simulink model "AC_System_with_Functions"  (R2021b)
settings: Solver=ode4  StartTime=0.0  StopTime=50  FixedStep=0.05  RelTol=1e-3
values from neighbouring files (symbols this model uses):
  ActiveMode =     [AC_System_Variables.mat]
  command =     [AC_System_Variables.mat]
  Fan_Input_Modes =     [AC_System_Variables.mat]
  FanModes =     [AC_System_Variables.mat]
  RequestedMode =     [AC_System_Variables.mat]
  state =     [AC_System_Variables.mat]
undefined symbols (not defined in the file or in its folder): sigbuilder_block
settings Model: Creator=t  LastModifiedBy=t

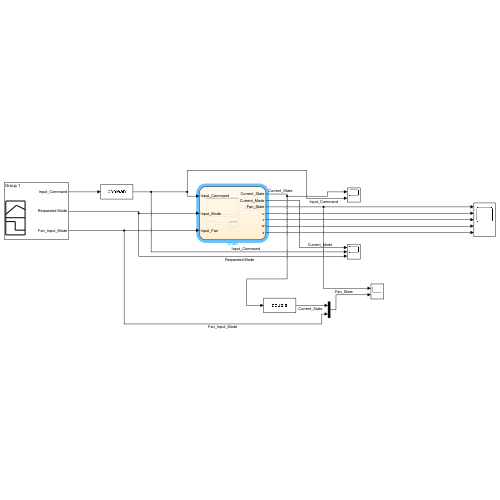
[thumbnail: Simulink's stored preview of the top-level diagram]
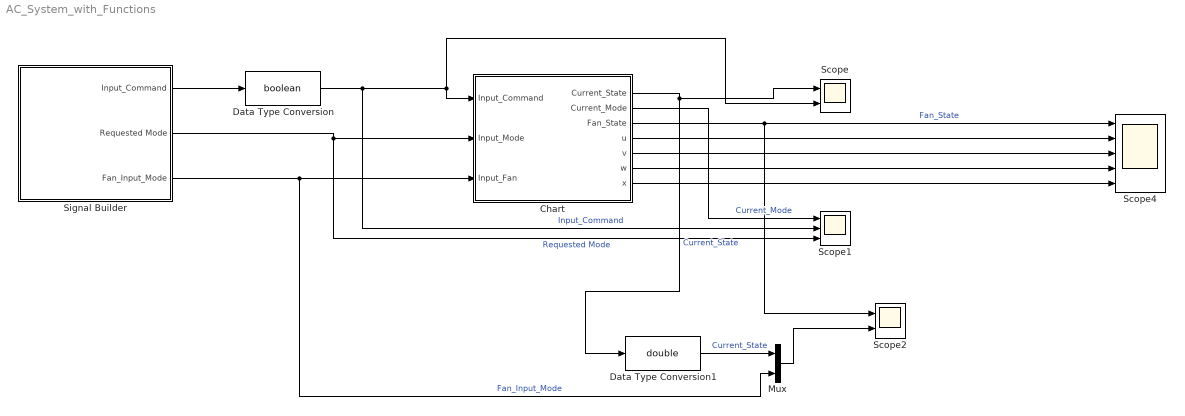
== system AC_System_with_Functions ==
  Chart : Stateflow chart  TreatAsAtomicUnit=on
  Data Type Conversion : DataTypeConversion  OutDataTypeStr=boolean
  Data Type Conversion1 : DataTypeConversion  OutDataTypeStr=double
  Mux : Mux  Inputs=2
  Scope : Scope  NumInputPorts=2
  Scope1 : Scope  NumInputPorts=3
  Scope2 : Scope  NumInputPorts=2
  Scope4 : Scope  NumInputPorts=5
  Signal Builder : Subsystem  Tag=STV Subsys  LoadFcn=sigbuilder_block('load');  StartFcn=sigbuilder_block('start');  StopFcn=sigbuilder_block('stop');  ClipboardFcn=sigbuilder_block('clipboard');  mask(Sigbuilder block){tuvar=[0:10]}
      mask help: Simulink:masks:SigbuilderBlock_MD
      mask init:
      | if ~strcmp(get_param(bdroot(gcbh),'SimulationStatus'),'stopped') tuvar = sigbuilder_block('maskInit'); end
      settings: CopyFcn=sigbuilder_block('copy');  DeleteFcn=sigbuilder_block('delete');  ModelCloseFcn=sigbuilder_block('modelClose');  PreSaveFcn=sigbuilder_block('preSave');  PauseFcn=sigbuilder_block('pause');  ContinueFcn=sigbuilder_block('continue');  NameChangeFcn=sigbuilder_block('namechange');  OpenFcn=sigbuilder_block('open',[5.4 30 1141.2 522.6 ]);  CloseFcn=sigbuilder_block('close');
      mask Display: plot(0, 0, 100, 100,[2, 2, 32, 32, 2], [68, 8, 8, 68, 68],[32, 2], [38, 38], [32, 19, 2],[53, 60, 44], [32, 17, 17, 2],[16, 16, 31, 31]);txt = getActiveGroup(gcbh);text(2, 100, txt,'verticalAlignment', 'top');
  wires:
  Signal Builder/1(Input_Command) -> Data Type Conversion/1
  Data Type Conversion/1 -> Scope1/2, Scope/2, Chart/1(Input_Command)  "Input_Command"
  Signal Builder/2(Requested Mode) -> Scope1/3, Chart/2(Input_Mode)  "Requested Mode"
  Chart/2(Current_Mode) -> Scope1/1  "Current_Mode"
  Chart/1(Current_State) -> Data Type Conversion1/1, Scope/1  "Current_State"
  Chart/3(Fan_State) -> Scope2/1, Scope4/1  "Fan_State"
  Signal Builder/3(Fan_Input_Mode) -> Mux/2, Chart/3(Input_Fan)  "Fan_Input_Mode"
  Mux/1 -> Scope2/2
  Data Type Conversion1/1 -> Mux/1  "Current_State"
  Chart/5(v) -> Scope4/3
  Chart/4(u) -> Scope4/2
  Chart/6(w) -> Scope4/4
  Chart/7(x) -> Scope4/5

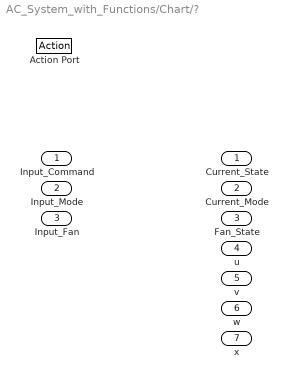
== system AC_System_with_Functions/Chart/? ==
  Input_Command : Inport
  Input_Mode : Inport  Port=2
  Input_Fan : Inport  Port=3
  Action Port : ActionPort
      settings: CopyFcn=Stateflow.SLINSF.SimulinkMan.removeBlockPreDeleteFcn  PreDeleteFcn=Stateflow.SLINSF.SimulinkMan.unsafePredeleteFcn
  Current_State : Outport
  Current_Mode : Outport  Port=2
  Fan_State : Outport  Port=3
  u : Outport  Port=4
  v : Outport  Port=5
  w : Outport  Port=6
  x : Outport  Port=7

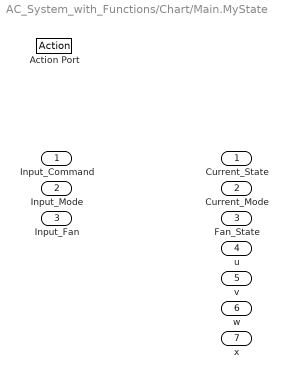
== system AC_System_with_Functions/Chart/Main.MyState ==
  Input_Command : Inport
  Input_Mode : Inport  Port=2
  Input_Fan : Inport  Port=3
  Action Port : ActionPort
      settings: CopyFcn=Stateflow.SLINSF.SimulinkMan.removeBlockPreDeleteFcn  PreDeleteFcn=Stateflow.SLINSF.SimulinkMan.unsafePredeleteFcn
  Current_State : Outport
  Current_Mode : Outport  Port=2
  Fan_State : Outport  Port=3
  u : Outport  Port=4
  v : Outport  Port=5
  w : Outport  Port=6
  x : Outport  Port=7

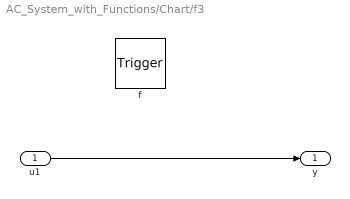
== system AC_System_with_Functions/Chart/f3 ==
  u1 : Inport  OutDataTypeStr=double  PortDimensions=1
  f : TriggerPort  TriggerType=function-call  VariantControl=(inherit)
      settings: CopyFcn=Stateflow.SLINSF.SimulinkMan.removeBlockPreDeleteFcn  PreDeleteFcn=Stateflow.SLINSF.SimulinkMan.unsafePredeleteFcn
  y : Outport
  wires:
  u1/1 -> y/1

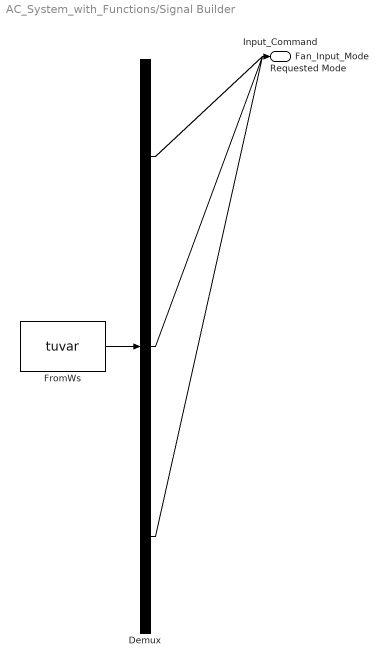
== system AC_System_with_Functions/Signal Builder ==
  Demux : Demux  Tag=STV Demux  Outputs=3
      settings: DisplayOption=none
  FromWs : FromWorkspace  Tag=STV FromWs  VariableName=tuvar
      SigBuilderData=|
      | common.afterFinalStr = 'Extrapolate'
      | common.sampleTime = 0
      | dataSet.timeRange = [0 50]
      | dataSet.name = 'Group 1'
      | sbobj.Groups.Name = 'Group 1'
      | sbobj.Groups.Signals(1).Name = 'Input_Command'
      | sbobj.Groups.Signals(1).XData = [0 1.3 1.3 33.5 33.5 36.5 36.5 38 38 40.2 40.2 47 47 50]
      | sbobj.Groups.Signals(1).YData = [0 0 1 1 0 0 1 1 0 0 1 1 0 0]
      | sbobj.Groups.Signals(2).Name = 'Requested Mode'
      | sbobj.Groups.Signals(2).XData = [0 2.5 2.5 4.55 4.55 7.25 7.25 17.4 17.4 28.2 28.2 38 38 44 44 50]
      | sbobj.Groups.Signals(2).YData = [0 0 1 1 2 2 4 4 2 2 4 4 3 3 2 2]
      | sbobj.Groups.Signals(3).Name = 'Fan_Input_Mode'
      | sbobj.Groups.Signals(3).XData = [0 5 5 20 20 35 35 44.95 44.95 45 50]
      | sbobj.Groups.Signals(3).YData = [1 1 3 3 2 2 3 3 1 1 1]
      | sbobj.Groups.TimeRange = [0 50]
  Input_Command : Outport  Tag=STV Outport
  Requested Mode : Outport  Tag=STV Outport  Port=2
  Fan_Input_Mode : Outport  Tag=STV Outport  Port=3
  wires:
  FromWs/1 -> Demux/1
  Demux/1 -> Input_Command/1
  Demux/2 -> Requested Mode/1
  Demux/3 -> Fan_Input_Mode/1

== stateflow chart AC_System_with_Functions/Chart ==
  state Main [parallel]
    settings: executionOrder=1
    state ON
      entry: Current_State=state.ON;
      (history)
      state Hot
        en: Current_Mode=ActiveMode.Hot;
        en: w=1;
        du: w=w+1;
        %ex: w=0;
        ex: v=2;
      state Cold
        en: Current_Mode=ActiveMode.Cold;
        en: u=1
        ex: u=0
      state Wet
        en: Current_Mode=ActiveMode.Wet;
        (default) -> (junction 107)
        Wet -> (junction 107) [order 1]
        (junction 107) -> (junction 108) [order 1] : [w>=80]
        (junction 108) -> (junction 109) : {w=5;}
        (junction 107) -> (junction 110) [order 2]
        (junction 110) -> (junction 120) [order 1] : [w==5]
        (junction 120) -> (junction 115) : {w=6;}
        (junction 110) -> (junction 118) [order 2]
      state Dry
        en: Current_Mode=ActiveMode.Dry;
      (default) -> Cold
      Hot -> Cold [order 1] : [Input_Mode==RequestedMode.Cold]
      Cold -> Hot [order 1] : [Input_Mode==RequestedMode.Hot]
      Cold -> Wet [order 3] : [Input_Mode==RequestedMode.Wet]
      Wet -> Cold [order 3] : [Input_Mode==RequestedMode.Cold]
      Dry -> Cold [order 2] : [Input_Mode==RequestedMode.Cold]
      Cold -> Dry [order 2] : [Input_Mode==RequestedMode.Dry]
      Hot -> Wet [order 3] : [Input_Mode==RequestedMode.Wet]
      Wet -> Hot [order 2] : [Input_Mode==RequestedMode.Hot]
      Dry -> Hot [order 1] : [Input_Mode==RequestedMode.Hot]
      Hot -> Dry [order 2] : [Input_Mode==RequestedMode.Dry]
      Wet -> Dry [order 1] : [Input_Mode==RequestedMode.Dry]
      Dry -> Wet [order 3] : [Input_Mode==RequestedMode.Wet]
    state MyState
    state OFF
      entry: Current_State=state.OFF;
      entry: Current_Mode=ActiveMode.Off;
      state OFF1
        en: x=1;
        ex: x=0;
      state OFF2
      (default) -> OFF1
      OFF1 -> OFF2
    OFF -> MyState [order 2] : [Input_Command==15]
    (default) -> OFF
    ON -> OFF : [hasChangedTo(Input_Command,command.OFF)]{send(GoOn,Fan);}
    OFF -> ON [order 1] : [hasChangedTo(Input_Command,command.ON)]{send(GoOff,Fan)}
  state y=f1(u1) [function]
    (default) -> (junction 159)
    (junction 159) -> (junction 164) [order 1] : [u1>5]
    (junction 164) -> (junction 166) : {x=19;y=55;}
    (junction 159) -> (junction 168) [order 2] : {y=50;}
  state y=f3(u1) [function]
  state ? [parallel]
    settings: executionOrder=3
  state Fan [parallel]
    settings: executionOrder=2
    state FanOFF
      en: Fan_State=FanModes.Off
    state FanON
      state Low
        en: Fan_State=FanModes.Low
        du: w=f1(v);
      state Med
        en: Fan_State=FanModes.Med
      state High
        en: Fan_State=FanModes.High
      Low -> (junction 132) [order 1] : [Input_Fan==Fan_Input_Modes.High]
      (junction 132) -> High
      (default) -> Low
      Med -> High [order 2] : [Input_Fan==Fan_Input_Modes.High]
      Low -> Med [order 2] : [Input_Fan==Fan_Input_Modes.Med]
      (junction 173) -> Low : [after(5,sec)]{x=1;}/{u=u+1;v=15}
      Med -> (junction 173) [order 1] : [Input_Fan==Fan_Input_Modes.Low]
      High -> Med [order 1] : [Input_Fan==Fan_Input_Modes.Med]
      High -> Low [order 2] : [Input_Fan==Fan_Input_Modes.Low]
    (default) -> FanOFF
    FanOFF -> FanON : GoOn
    FanON -> FanOFF : GoOff
  data: sf_internal_action_state_placeholder_data local double size=1 =0; u1 function_input; y function_output; u1 function_input; y function_output; y2 function_output; u1 function_input double size=1; y function_output; sf_internal_action_state_placeholder_data local double size=1 =0; Input_Command input; Current_State output; command parameter; state parameter; counter local uint8 =uint8(0); limit constant uint8 =20; Current_Mode output =0; RequestedMode parameter; ActiveMode parameter; Input_Mode input; Input_Fan input; Fan_State output; FanModes parameter; Fan_Input_Modes parameter; Main_State local boolean =false; ON constant boolean =true; OFF constant boolean =false; u output; v output; w output; x output
  events: GoOn local FUNCTION_CALL_EVENT; GoOff local FUNCTION_CALL_EVENT
  function [y,y2]=f2(u1):
    | function [y,y2]=f2(u1)
    |  if u1>5
    |      y=55;
    |      y2=19;
    |  else
    |      y=50;
    |      y2=0;
    |  end
